simulink model "quadrotor_demo"  (Simulink 7.5)
settings: Solver=ode45  StartTime=0.0  StopTime=100  RelTol=1e-3
undefined symbols (not defined in the file): STARMAC, uav_utilities
libraries: aero_sim_lib x8, simulink x1
(part 2 of 2)

== matlab function STARMAC/gum_stix/sensor_fusion/FuseData ==
  data: Xe_s input single size=[3]; out_data output single; Xe_f input single size=[3]; Ve_s input single size=[3]; Ve_f input single size=[3]; dV_1p input double; dX_1p input double; Ve_sh_1p input double; Xe_sh_1p input double
function out_data  = fcn(Xe_s, Xe_f, Ve_s, Ve_f,dV_1p,dX_1p,Ve_sh_1p,Xe_sh_1p)
%function [Xe,Ve,dV_1,dX_1,Ve_sh_1,Xe_sh_1] = fcn(Xe_s, Xe_f, Ve_s, Ve_f,dV_1p,dX_1p,Ve_sh_1p,Xe_sh_1p)
%#eml

%persistent dV_1p dX_1p Ve_sh_1p Xe_sh_1p

%if ( isempty( dV_1p ) )
%   dV_1p = zeros(size(Ve_s),'single');
%   dX_1p = zeros(size(Xe_s),'single');
%   Ve_sh_1p = dV_1p;
%   Xe_sh_1p = dX_1p;
%end

if ((Xe_s(1) ~= Xe_sh_1p(1)) || (Xe_s(2) ~= Xe_sh_1p(2)) || (Xe_s(3) ~= Xe_sh_1p(3)))
    Xe_sh_1 = Xe_s;
    dX_1 = Xe_f - Xe_s;
else
    Xe_sh_1 = Xe_sh_1p;
    dX_1 = dX_1p;
end


if ((Ve_s(1) ~= Ve_sh_1p(1)) || (Ve_s(2) ~= Ve_sh_1p(2)) || (Ve_s(3) ~= Ve_sh_1p(3)))
    Ve_sh_1 = Ve_s;
    dV_1 = Ve_f - Ve_s;
else
    Ve_sh_1 = Ve_sh_1p;
    dV_1 = dV_1p;
end

%dV_1p = dV_1;
%dX_1p = dX_1;
%Ve_sh_1p = Ve_sh_1;
%Xe_sh_1p = Xe_sh_1;

Xe = Xe_f - dX_1;
Ve = Ve_f - dV_1;

out_data = [Xe; Ve; dV_1; dX_1; Ve_sh_1; Xe_sh_1 ];

== matlab function STARMAC/gum_stix/inertial_pos_controller/demux_fc_xyz ==
  data: fc_xyz input single size=[3]; fc_x output single size=[1]; fc_y output single size=[1]; fc_z output single size=[1]
function [fc_x,fc_y, fc_z] = fcn(fc_xyz)
% This block supports the Embedded MATLAB subset.
% See the help menu for details. 
fc_x=fc_xyz(1);
fc_y=fc_xyz(2);
fc_z=fc_xyz(3);

== matlab function STARMAC/gum_stix/inertial_pos_controller/mux_euler ==
  data: ficx_ficz input single size=[1]; euler output single size=[3]; ficy_ficz input single size=[1]; psi_a input single size=[1]; psi_s input single size=[1]
function euler = fcn(ficx_ficz, ficy_ficz, psi_a, psi_s)
% This block supports the Embedded MATLAB subset.
% See the help menu for details. 

A = [sin(psi_a) -cos(psi_a); cos(psi_a) sin(psi_a)];
% Get [phi, theta] 
euler_angs = (A * [ficx_ficz; ficy_ficz])';

euler=[euler_angs(1);euler_angs(2);psi_s];

== matlab function STARMAC/gum_stix/rate_limiter/Embedded MATLAB Function ==
  data: Xd input single size=[3]; Xr output single; Xd_prev input single size=[3]; Tsamp input single size=[1]; Vmax input single size=[1]
function Xr = limit_rate(Xd, Xd_prev, Tsamp, Vmax)
% This block supports the Embedded MATLAB subset.
% See the help menu for details. 

delta = Xd - Xd_prev;
delta = sign(delta) .* min( abs(delta), (ones(3,1) * Tsamp * Vmax) );

Xr = Xd_prev + delta;

== matlab function STARMAC/robo_stix/inner_loop/u_T_u_torque_motor_thrust/u_torque_u_T_mux ==
  data: u_torque input single size=[3]; u_torque_u_T output single size=[4]; u_T input single size=[1]
function u_torque_u_T = fcn(u_torque, u_T)
% This block supports the Embedded MATLAB subset.
% See the help menu for details. 
u_torque_u_T = [u_torque; u_T];
